simulink model "blockdemo"  (Simulink 6.3)
settings: Solver=FixedStepDiscrete  StartTime=0.0  StopTime=10.0  FixedStep=1  RelTol=1e-3
InitFcn:
  | %% DSPBuilder Start
  | alt_dspbuilder_update_model(bdroot)
  | %% DSPBuilder End
libraries: allblocks_alteradspbuilder2 x4
settings Model: LastModifiedBy=LKONG

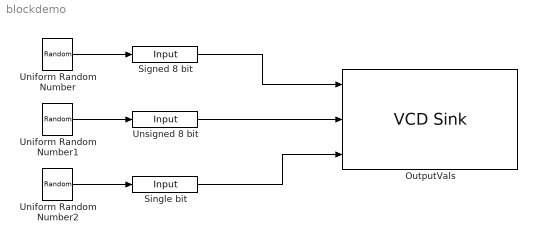
== system blockdemo ==
  OutputVals : allblocks_alteradspbuilder2/VCD Sink  inNames=Port1 Port2 Port3  inBwls=0 0 0  inBwrs=0 0 0  inTypes=i i i  inDelayed=1 1 1  Inputs=3  TextFilePath=d:\wsTrunk\workspace\Documentation\DesignExamples\Tutorials\UnitBlocks\AltLab\VCDSink\OutputVals.txt
  Signed 8 bit : allblocks_alteradspbuilder2/Input  iofile=d:\wsTrunk\workspace\Documentation\DesignExamples\Tutorials\UnitBlocks\AltLab\VCDSink\tb_blockdemo\blockdemo_Signed+8+bit.salt  BusType=Signed Integer  bwl=8  bwr=8  SpecifyClock=off  PORTTYPE=Input
  Single bit : allblocks_alteradspbuilder2/Input  iofile=d:\wsTrunk\workspace\Documentation\DesignExamples\Tutorials\UnitBlocks\AltLab\VCDSink\tb_blockdemo\blockdemo_Single+bit.salt  BusType=Single Bit  bwl=8  bwr=8  SpecifyClock=off  PORTTYPE=Input
  Uniform Random Number : UniformRandomNumber  Minimum=-128  Maximum=127  SampleTime=0
  Uniform Random Number1 : UniformRandomNumber  Minimum=0  Maximum=255  SampleTime=0
  Uniform Random Number2 : UniformRandomNumber  Minimum=0  SampleTime=0
  Unsigned 8 bit : allblocks_alteradspbuilder2/Input  iofile=d:\wsTrunk\workspace\Documentation\DesignExamples\Tutorials\UnitBlocks\AltLab\VCDSink\tb_blockdemo\blockdemo_Unsigned+8+bit.salt  BusType=Signed Integer  bwl=8  bwr=8  SpecifyClock=off  PORTTYPE=Input
  wires:
  Signed 8 bit/1 -> OutputVals/1
  Unsigned 8 bit/1 -> OutputVals/2
  Single bit/1 -> OutputVals/3
  Uniform Random Number/1 -> Signed 8 bit/1
  Uniform Random Number1/1 -> Unsigned 8 bit/1
  Uniform Random Number2/1 -> Single bit/1
